simulink model "KaplunenkoDD_Task3"  (R2020a)
settings: Solver=VariableStepAuto  StartTime=0.0  StopTime=100  RelTol=1e-3  EnableMultiTasking=on
libraries: simulink x9
settings Model: Creator=Boris  LastModifiedBy=Dmitry Kaplunenko
settings DataIOCC: SaveOutput=off  SignalLogging=off  DSMLogging=off  SaveTime=off  ReturnWorkspaceOutputs=off
settings OptimizationCC: LifeSpan=inf
settings DebuggingCC: SFUnexpectedBacktrackingDiag=warning  SFNoUnconditionalDefaultTransitionDiag=warning  SFExecutionAtInitializationDiag=none  ArithmeticOperatorsInVariantConditions=warning
settings SFSimCC: SimUseLocalCustomCode=off  CustomCodeUndefinedFunction=UseInterfaceOnly
settings RTWCC: RTWUseLocalCustomCode=off
settings CodeAppCC: StateflowObjectComments=on
settings GRTTargetCC: TargetLangStandard=C89/C90 (ANSI)
settings ConfigComp: CovMetricSettings=dw  CovHtmlReporting=on  CovSaveCumulativeToWorkspaceVar=on  CovSaveSingleToWorkspaceVar=on  CovExternalEMLEnable=off

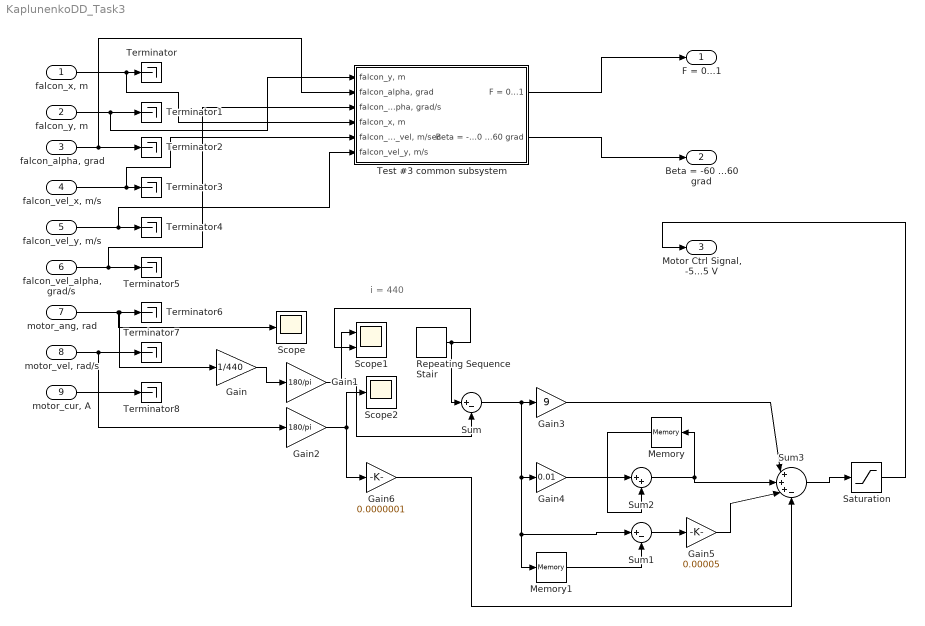
== system KaplunenkoDD_Task3 ==
  note: i = 440
  "falcon_x, m" : Inport  OutDataTypeStr=double  PortDimensions=1  SampleTime=[0.01,0]
  "falcon_y, m" : Inport  Port=2  OutDataTypeStr=double  PortDimensions=1  SampleTime=[0.01,0]
  "falcon_alpha, grad" : Inport  Port=3  OutDataTypeStr=double  PortDimensions=1  SampleTime=[0.01,0]
  "falcon_vel_x, m/s" : Inport  Port=4  OutDataTypeStr=double  PortDimensions=1  SampleTime=[0.01,0]
  "falcon_vel_y, m/s" : Inport  Port=5  OutDataTypeStr=double  PortDimensions=1  SampleTime=[0.01,0]
  "falcon_vel_alpha, grad/s" : Inport  Port=6  OutDataTypeStr=double  PortDimensions=1  SampleTime=[0.01,0]
  "motor_ang, rad" : Inport  Port=7  OutDataTypeStr=double  PortDimensions=1  SampleTime=[0.01,0]
  "motor_vel, rad/s" : Inport  Port=8  OutDataTypeStr=double  PortDimensions=1  SampleTime=[0.01,0]
  "motor_cur, A" : Inport  Port=9  OutDataTypeStr=double  PortDimensions=1  SampleTime=[0.01,0]
  Gain : Gain  Gain=1/440
  Gain1 : Gain  Gain=180/pi
  Gain2 : Gain  Gain=180/pi
  Gain3 : Gain  Gain=9
  Gain4 : Gain  Gain=0.01
  Gain5 : Gain  Gain=0.00005
  Gain6 : Gain  Gain=0.0000001
  Memory : Memory
  Memory1 : Memory
  Repeating Sequence Stair : simulink/Sources/Repeating Sequence Stair  OutValues=[90 110 135].'  tsamp=15  OutMin=[]  OutMax=[]  OutDataTypeStr=double  OutputDataTypeScalingMode=double  OutDataType=fixdt(0,8)  ConRadixGroup=Best Precision: Vector-wise  OutScaling=2^-12
  Saturation : Saturate  UpperLimit=5  LowerLimit=-5
  Scope : Scope
  Scope1 : Scope  NumInputPorts=2
  Scope2 : Scope
  Sum : Sum  Inputs=|+-
  Sum1 : Sum  Inputs=|+-
  Sum2 : Sum  Inputs=|++
  Sum3 : Sum  Inputs=|+++-
  Terminator{,1..8} (9 alike) : Terminator
  Test #3 common subsystem : Subsystem
  F = 0...1 : Outport  OutDataTypeStr=double  PortDimensions=1  SampleTime=[0.01,0]  VectorParamsAs1DForOutWhenUnconnected=off
  Beta = -60 ...60 grad : Outport  Port=2  OutDataTypeStr=double  PortDimensions=1  SampleTime=[0.01,0]  VectorParamsAs1DForOutWhenUnconnected=off
  "Motor Ctrl Signal, -5...5 V" : Outport  Port=3  OutDataTypeStr=double  PortDimensions=1  SampleTime=[0,1]  VectorParamsAs1DForOutWhenUnconnected=off
  wires:
  "motor_ang, rad"/1 -> Scope/1, Terminator6/1, Gain/1
  "falcon_vel_y, m/s"/1 -> Terminator4/1, Test #3 common subsystem/6("falcon_vel_y, m/s")
  "falcon_vel_x, m/s"/1 -> Terminator3/1, Test #3 common subsystem/5("falcon_x_vel, m/sec")
  "falcon_alpha, grad"/1 -> Terminator2/1, Test #3 common subsystem/2("falcon_alpha, grad")
  "falcon_y, m"/1 -> Terminator1/1, Test #3 common subsystem/1("falcon_y, m")
  "falcon_x, m"/1 -> Terminator/1, Test #3 common subsystem/4("falcon_x, m")
  "motor_vel, rad/s"/1 -> Terminator7/1, Gain2/1
  "motor_cur, A"/1 -> Terminator8/1
  "falcon_vel_alpha, grad/s"/1 -> Terminator5/1, Test #3 common subsystem/3("falcon_vel_alpha, grad/s")
  Gain/1 -> Gain1/1
  Gain1/1 -> Scope1/1, Sum/2
  Gain2/1 -> Scope2/1, Gain6/1
  Repeating Sequence Stair/1 -> Scope1/2, Sum/1
  Sum/1 -> Gain3/1, Gain4/1, Memory1/1, Sum1/1
  Gain4/1 -> Sum2/1
  Gain3/1 -> Sum3/1
  Sum2/1 -> Sum3/2, Memory/1
  Memory/1 -> Sum2/2
  Memory1/1 -> Sum1/2
  Sum1/1 -> Gain5/1
  Gain5/1 -> Sum3/3
  Sum3/1 -> Saturation/1
  Saturation/1 -> "Motor Ctrl Signal, -5...5 V"/1
  Gain6/1 -> Sum3/4
  Test #3 common subsystem/2(Beta = -60 ...60 grad) -> Beta = -60 ...60 grad/1
  Test #3 common subsystem/1(F = 0...1) -> F = 0...1/1

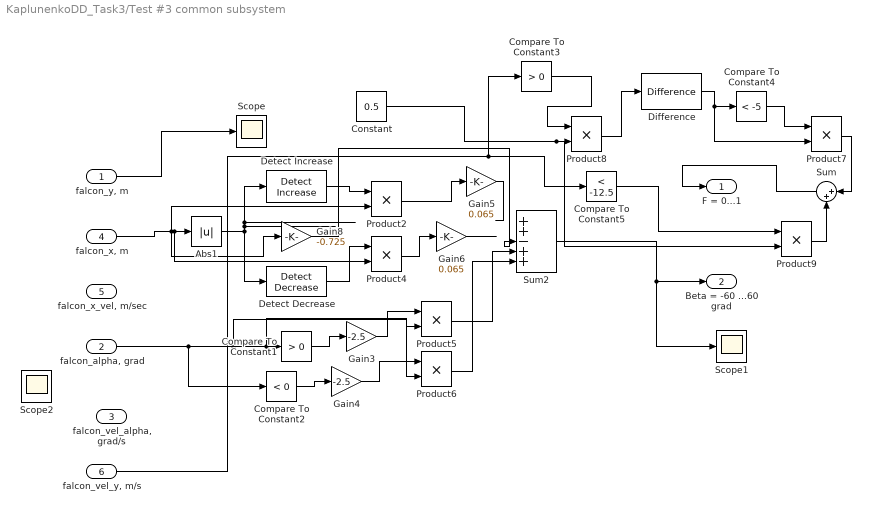
== system KaplunenkoDD_Task3/Test #3 common subsystem ==
  "falcon_y, m" : Inport
  "falcon_alpha, grad" : Inport  Port=2
  "falcon_vel_alpha, grad/s" : Inport  Port=3
  "falcon_x, m" : Inport  Port=4
  "falcon_x_vel, m/sec" : Inport  Port=5
  "falcon_vel_y, m/s" : Inport  Port=6
  Abs1 : Abs
  Compare To Constant1 : simulink/Logic and Bit Operations/Compare To Constant  relop=>  const=0  OutDataTypeStr=boolean
  Compare To Constant2 : simulink/Logic and Bit Operations/Compare To Constant  relop=<  const=0  OutDataTypeStr=boolean
  Compare To Constant3 : simulink/Logic and Bit Operations/Compare To Constant  relop=>  const=0  OutDataTypeStr=boolean
  Compare To Constant4 : simulink/Logic and Bit Operations/Compare To Constant  relop=<  const=-5  OutDataTypeStr=boolean
  Compare To Constant5 : simulink/Logic and Bit Operations/Compare To Constant  relop=<  const=-12.5  OutDataTypeStr=boolean
  Constant : Constant  Value=0.5
  Detect Decrease : simulink/Logic and Bit Operations/Detect Decrease  vinit=0.0  OutDataTypeStr=boolean
  Detect Increase : simulink/Logic and Bit Operations/Detect Increase  vinit=0.0  OutDataTypeStr=boolean
  Difference : simulink/Discrete/Difference  ICPrevInput=0.0  OutMin=[]  OutMax=[]  OutDataType=fixdt(1, 16)  OutScaling=2^-10  DoSatur=off
  Gain3 : Gain  Gain=-2.5
  Gain4 : Gain  Gain=-2.5
  Gain5 : Gain  Gain=0.065
  Gain6 : Gain  Gain=0.065
  Gain8 : Gain  Gain=-0.725
  Product{2,4..9} (7 alike) : Product
  Scope : Scope
  Scope1 : Scope
  Scope2 : Scope
  Sum : Sum  Inputs=|++
  Sum2 : Sum  Inputs=|++-++
  F = 0...1 : Outport  VectorParamsAs1DForOutWhenUnconnected=off
  Beta = -60 ...60 grad : Outport  Port=2  VectorParamsAs1DForOutWhenUnconnected=off
  wires:
  Gain8/1 -> Sum2/3
  Sum/1 -> F = 0...1/1
  Product9/1 -> Sum/2
  Compare To Constant5/1 -> Product9/1
  Product8/1 -> Difference/1
  Product7/1 -> Sum/1
  Compare To Constant4/1 -> Product7/1
  Difference/1 -> Compare To Constant4/1, Product7/2
  Compare To Constant3/1 -> Product8/1
  "falcon_vel_y, m/s"/1 -> Compare To Constant3/1, Compare To Constant5/1
  Gain6/1 -> ?
  Gain5/1 -> ?
  Product6/1 -> Sum2/5
  Gain4/1 -> Product6/1
  Compare To Constant2/1 -> Gain4/1
  Gain3/1 -> Product5/1
  Product5/1 -> Sum2/4
  Compare To Constant1/1 -> Gain3/1
  Product4/1 -> Gain6/1
  Detect Decrease/1 -> Product4/1
  Sum2/1 -> Beta = -60 ...60 grad/1, Scope1/1
  Product2/1 -> Gain5/1
  Detect Increase/1 -> Product2/1
  Abs1/1 -> Detect Decrease/1, Detect Increase/1
  "falcon_x, m"/1 -> Abs1/1, Product4/2, Product2/2, Gain8/1
  "falcon_y, m"/1 -> Scope/1
  Constant/1 -> Product8/2, Product9/2
  "falcon_alpha, grad"/1 -> Compare To Constant1/1, Product6/2, Product5/2, Compare To Constant2/1
